simulink model "FuzzyHYPFWMLI"  (R2020b)
settings: Solver=ode23t  StartTime=0.0  StopTime=1  FixedStep=1.0000000100000003E-5  MaxStep=1e-3  RelTol=1e-2  EnableMultiTasking=on
undefined symbols (not defined in the file): c1, c2, c3, c4, c5, c6, DiscIntNeverNeededParam, FC1, FC2, idq1, idq2, PV10k1, PV10k2, PV10k3, R, WM1
libraries: powerlib x93, powerlib_meascontrol x9, fuzblock x8, powerlib_extras x6, re_lib x3, electricdrivelib x2, pid_lib x1
(part 1 of 2)
settings Model: Creator=yaju
settings SolverCC: ZeroCrossControl=DisableAll  AlgebraicLoopSolver=LineSearch
settings DataIOCC: ReturnWorkspaceOutputs=off
settings OptimizationCC: LifeSpan=inf
settings DebuggingCC: SFUnexpectedBacktrackingDiag=warning  SFNoUnconditionalDefaultTransitionDiag=warning  SFExecutionAtInitializationDiag=none  ArithmeticOperatorsInVariantConditions=warning
settings SFSimCC: SimUseLocalCustomCode=off  CustomCodeUndefinedFunction=UseInterfaceOnly
settings RTWCC: RTWUseLocalCustomCode=off
settings CodeAppCC: StateflowObjectComments=on
settings GRTTargetCC: TargetLangStandard=C89/C90 (ANSI)
settings ConfigComp: CovMetricSettings=dw  CovSaveCumulativeToWorkspaceVar=on  CovSaveSingleToWorkspaceVar=on  CovExternalEMLEnable=off  CovBoundaryAbsTol=1.0e-5
settings SimscapeCC: SimscapeNormalizeSystem=off

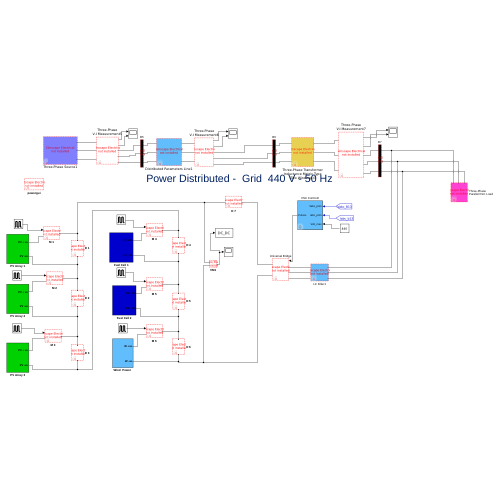
[thumbnail: Simulink's stored preview of the top-level diagram]
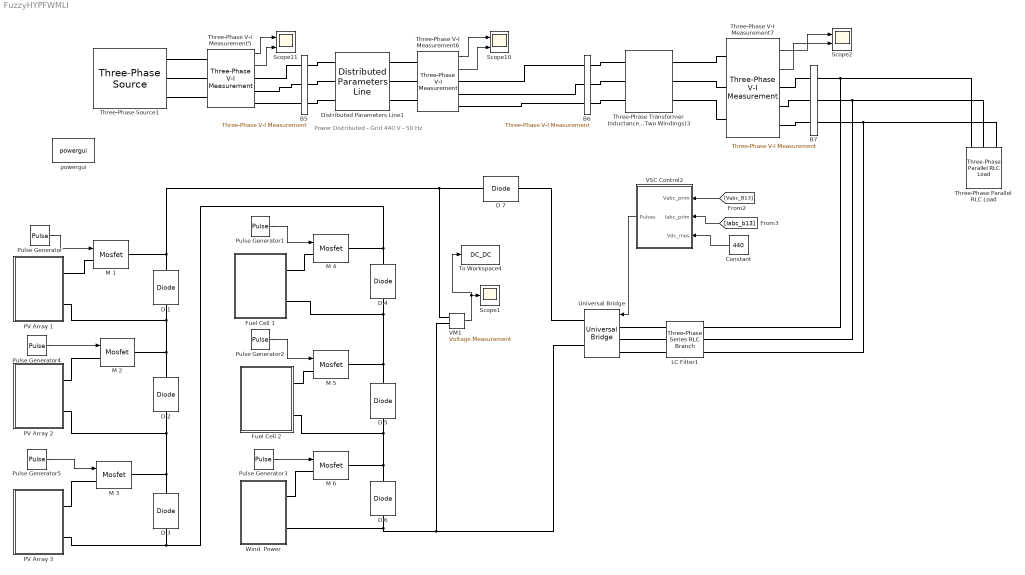
== system FuzzyHYPFWMLI ==
  note: Power Distributed - Grid 440 V - 50 Hz
  B5 : powerlib/Measurements/Three-Phase V-I Measurement  VoltageMeasurement=no  SetLabelV=off  LabelV=Vabc_B12  Vpu=off  VpuLL=off  CurrentMeasurement=no  SetLabelI=off  LabelI=A1  Ipu=off  Pbase=100e6  Vbase=25e3  OutputType=Magnitude  PhasorSimulation=off  PSBequivalent=0
  B6 : powerlib/Measurements/Three-Phase V-I Measurement  VoltageMeasurement=no  SetLabelV=off  LabelV=Vabc_B12  Vpu=off  VpuLL=off  CurrentMeasurement=no  SetLabelI=off  LabelI=A1  Ipu=off  Pbase=100e6  Vbase=440  OutputType=Magnitude  PhasorSimulation=off  PSBequivalent=0
  B7 : powerlib/Measurements/Three-Phase V-I Measurement  VoltageMeasurement=phase-to-ground  SetLabelV=on  LabelV=Vabc_B13  Vpu=off  VpuLL=off  CurrentMeasurement=yes  SetLabelI=on  LabelI=Iabc_b13  Ipu=off  Pbase=100e6  Vbase=440  OutputType=Magnitude  PhasorSimulation=off  PSBequivalent=0
  Constant : Constant  Value=440
  D {1..7} (7 alike) : powerlib/Power Electronics/Diode  Ron=0.00001  Lon=0  Vf=0  IC=0  UseSnubber=off  Rs=inf  Cs=0  Measurements=off
  Distributed Parameters Line1 : powerlib/Elements/Distributed Parameters Line  Phases=3  Frequency=50  Resistance=[0.01273 0.3864]  Inductance="[0.9337e-3  4.1264e-3]"  Capacitance=[12.74e-9 7.751e-9]  Length=100  x1=[-0.00057 -1.30078134445774e-10 0 0;-0.00056 -1.32375687672932e-10 0 0;-0.00055 -1.34671934405495e-10 0 0;-0.00054 -1.36966851980434e-10 0 0;-0.00053 -1.3926041774784e-10 0 0;-0.00052 -1.41552609071144e-10 0 0;-0.00051 -1.43843403327344e-10 0 0;-0.0005 -1.46132777907226e-10 0 0;-0.00049 -1.48420710215585e-10 0 0;-0.00048 -1.50707177671454e-10 0 0;-0.00047 -1.52992157708323e-10 0 0;-0.00046 -1.55275627774361e-10 0 0;-0.00045 -1.5755756533264e-10 0 0;-0.00044 -1.59837947861357e-10 0 0;-0.00043 -1.62116752854058e-10 0 0;-0.00042 -1.64393957819858e-10 0 0;-0.00041 -1.66669540283663e-10 0 0;-0.0004 -1.68943477786392e-10 0 0;-0.00039 -1.71215747885201e-10 0 0;-0.00038 -1.73486328153701e-10 0 0;-0.00037 -1.75755196182181e-10 0 0;-0.00036 -1.7802232957783e-10 0 0;-0.00035 -1.80287705964957e-10 25764.9329895724 -59181.0282967784;-0.00034 -1.82551302985211e-10 25950.7282227276 -59099.7934592953;-0.00033 -1.84813098297803e-10 26136.267332672 -59017.9753307104;-0.00032 -1.87073069579727e-10 26321.5484882094 -58935.5747185355;-0.00031 -1.89331194525979e-10 26506.5698606897 -58852.5924360314;-0.0003 -1.91587450849777e-10 26691.3296240266 -58769.0293021996;-0.00029 -1.93841816282782e-10 26875.8259547158 -58684.8861417747;-0.00028 -1.96094268575318e-10 27060.0570318531 -58600.1637852156;-0.00027 -1.98344785496589e-10 27244.0210371521 -58514.8630686978;-0.00026 -2.00593344834902e-10 27427.7161549622 -58428.9848341049;-0.00025 -2.02839924397885e-10 27611.140572287 -58342.5299290204;-0.00024 -2.05084502012703e-10 27794.2924788014 -58255.4992067194;-0.00023 -2.07327055526283e-10 27977.17006687 -58167.8935261599;-0.00022 -2.09567562805526e-10 28159.7715315649 -58079.7137519746;-0.00021 -2.1180600173753e-10 28342.0950706833 -57990.9607544623;-0.0002 -2.14042350229806e-10 28524.1388847655 -57901.6354095792;-0.00019 -2.16276586210498e-10 28705.9011771127 -57811.7385989305;-0.00018 -2.18508687628599e-10 28887.3801538042 -57721.2712097614;-0.00017 -2.20738632454168e-10 29068.5740237159 -57630.2341349485;-0.00016 -2.2296639867855e-10 29249.4809985375 -57538.6282729909;-0.00015 -2.25191964314593e-10 29430.0992927901 -57446.4545280015;-0.00014 -2.27415307396862e-10 29610.4271238441 -57353.713809698;-0.00013 -2.29636405981858e-10 29790.4627119366 -57260.4070333939;-0.00012 -2.31855238148235e-10 29970.2042801891 -57166.5351199893;-0.00011 -2.34071781997015e-10 30149.6500546247 -57072.0989959621;-0.0001 -2.36286015651805e-10 30328.7982641862 -56977.0995933588;-9e-05 -2.38497917259013e-10 30507.6471407531 -56881.537849785;-8e-05 -2.40707464988064e-10 30686.1949191592 -56785.4147083967;-7e-05 -2.42914637031613e-10 30864.4398372099 -56688.7311178905;-6e-05 -2.45119411605762e-10 31042.3801356999 -56591.4880324942;-5e-05 -2.47321766950278e-10 31220.0140584302 -56493.686411958;-4e-05 -2.49521681328802e-10 31397.3398522259 -56395.3272215443;-3e-05 -2.51719133029067e-10 31574.3557669528 -56296.4114320187;-2e-05 -2.53914100363113e-10 31751.0600555354 -56196.94001964;-1e-05 -2.56106561667497e-10 31927.4509739736 -56096.9139661509]  x2=[-0.00057 -2.06840243965178e-10 0 0;-0.00056 -2.16852614078585e-10 0 0;-0.00055 -2.26862843944237e-10 0 0;-0.00054 -2.36870834765207e-10 0 0;-0.00053 -2.46876487766668e-10 0 0;-0.00052 -2.56879704196862e-10 0 0;-0.00051 -2.66880385328082e-10 0 0;-0.0005 -2.76878432457643e-10 0 0;-0.00049 -2.86873746908856e-10 0 0;-0.00048 -2.96866230032002e-10 0 0;-0.00047 -3.06855783205308e-10 0 0;-0.00046 -3.16842307835916e-10 0 0;-0.00045 -3.2682570536086e-10 0 0;-0.00044 -3.36805877248038e-10 0 0;-0.00043 -3.46782724997181e-10 0 0;-0.00042 -3.5675615014083e-10 0 0;-0.00041 -3.66726054245305e-10 0 0;-0.0004 -3.76692338911678e-10 0 0;-0.00039 -3.86654905776744e-10 0 0;-0.00038 -3.96613656513988e-10 0 0;-0.00037 -4.06568492834561e-10 0 0;-0.00036 -4.16519316488249e-10 0 0;-0.00035 -4.26466029264439e-10 25871.2785310306 -59545.5888484983;-0.00034 -4.36408532993091e-10 26058.2185382591 -59464.0181181603;-0.00033 -4.46346729545707e-10 26244.9013613908 -59381.8605019701;-0.00032 -4.56280520836301e-10 26431.3251579416 -59299.1168107902;-0.00031 -4.66209808822362e-10 26617.4880879838 -59215.7878612673;-0.0003 -4.76134495505826e-10 26803.3883141644 -59131.8744758247;-0.00029 -4.86054482934043e-10 26989.0240017234 -59047.3774826534;-0.00028 -4.95969673200741e-10 27174.3933185114 -58962.2977157048;-0.00027 -5.05879968446996e-10 27359.4944350081 -58876.6360146818;-0.00026 -5.15785270862194e-10 27544.3255243402 -58790.3932250308;-0.00025 -5.25685482685e-10 27728.8847622995 -58703.5701979333;-0.00024 -5.3558050620432e-10 27913.1703273608 -58616.1677902975;-0.00023 -5.45470243760266e-10 28097.1804006999 -58528.18686475;-0.00022 -5.55354597745121e-10 28280.9131662118 -58439.6282896269;-0.00021 -5.65233470604303e-10 28464.3668105282 -58350.4929389656;-0.0002 -5.75106764837323e-10 28647.5395230356 -58260.781692496;-0.00019 -5.84974382998755e-10 28830.4294958935 -58170.495435632;-0.00018 -5.9483622769919e-10 29013.0349240516 -58079.6350594623;-0.00017 -6.04692201606202e-10 29195.354005268 -57988.2014607424;-0.00016 -6.14542207445309e-10 29377.384940127 -57896.1955418848;-0.00015 -6.24386148000929e-10 29559.1259320568 -57803.6182109509;-0.00014 -6.34223926117344e-10 29740.5751873472 -57710.4703816414;-0.00013 -6.44055444699654e-10 29921.7309151672 -57616.752973288;-0.00012 -6.5388060671474e-10 30102.5913275829 -57522.4669108435;-0.00011 -6.63699315192221e-10 30283.1546395752 -57427.6131248734;-0.0001 -6.73511473225407e-10 30463.419069057 -57332.1925515463;-9e-05 -6.8331698397226e-10 30643.3828368911 -57236.2061326245;-8e-05 -6.93115750656347e-10 30823.0441669079 -57139.6548154555;-7e-05 -7.02907676567797e-10 31002.4012859225 -57042.5395529616;-6e-05 -7.12692665064255e-10 31181.4524237526 -56944.8613036313;-5e-05 -7.22470619571835e-10 31360.1958132358 -56846.6210315096;-4e-05 -7.32241443586072e-10 31538.6296902468 -56747.8197061882;-3e-05 -7.42005040672879e-10 31716.7522937155 -56648.4583027963;-2e-05 -7.51761314469494e-10 31894.5618656437 -56548.5378019908;-1e-05 -7.61510168685434e-10 32072.0566511226 -56448.0591899468]  x3=[-0.00057 1.68975280202087e-11 0 0;-0.00056 1.68765883509604e-11 0 0;-0.00055 1.68554821165985e-11 0 0;-0.00054 1.68342095254328e-11 0 0;-0.00053 1.68127707874154e-11 0 0;-0.00052 1.67911661141379e-11 0 0;-0.00051 1.67693957188297e-11 0 0;-0.0005 1.67474598163559e-11 0 0;-0.00049 1.67253586232149e-11 0 0;-0.00048 1.67030923575366e-11 0 0;-0.00047 1.668066123908e-11 0 0;-0.00046 1.66580654892313e-11 0 0;-0.00045 1.66353053310013e-11 0 0;-0.00044 1.66123809890236e-11 0 0;-0.00043 1.65892926895523e-11 0 0;-0.00042 1.65660406604595e-11 0 0;-0.00041 1.65426251312333e-11 0 0;-0.0004 1.65190463329757e-11 0 0;-0.00039 1.64953044983997e-11 0 0;-0.00038 1.64713998618278e-11 0 0;-0.00037 1.6447332659189e-11 0 0;-0.00036 1.64231031280169e-11 0 0;-0.00035 1.63987115074472e-11 70.7662938963626 -227.139574442311;-0.00034 1.63741580382154e-11 71.479523523603 -226.916135051034;-0.00033 1.63494429626542e-11 72.1920476768036 -226.690456089114;-0.00032 1.63245665246915e-11 72.9038593236387 -226.462539783912;-0.00031 1.62995289698478e-11 73.6149514388149 -226.232388384868;-0.0003 1.62743305452334e-11 74.3253170041398 -226.000004163484;-0.00029 1.62489714995469e-11 75.0349490085923 -225.7653894133;-0.00028 1.62234520830715e-11 75.7438404483909 -225.528546449867;-0.00027 1.61977725476738e-11 76.4519843270633 -225.28947761073;-0.00026 1.61719331468004e-11 77.1593736555153 -225.048185255402;-0.00025 1.61459341354757e-11 77.8660014520998 -224.804671765341;-0.00024 1.61197757702994e-11 78.5718607426858 -224.558939543928;-0.00023 1.60934583094441e-11 79.276944560727 -224.310991016439;-0.00022 1.60669820126525e-11 79.9812459473307 -224.060828630027;-0.00021 1.60403471412349e-11 80.6847579513268 -223.808454853693;-0.0002 1.60135539580668e-11 81.3874736293355 -223.553872178265;-0.00019 1.5986602727586e-11 82.089386045837 -223.297083116371;-0.00018 1.59594937157904e-11 82.7904882732391 -223.038090202415;-0.00017 1.59322271902349e-11 83.4907733919458 -222.776895992553;-0.00016 1.59048034200292e-11 84.1902344904257 -222.513503064667;-0.00015 1.58772226758347e-11 84.8888646652801 -222.247914018337;-0.00014 1.58494852298623e-11 85.5866570213113 -221.980131474821;-0.00013 1.58215913558694e-11 86.2836046715904 -221.710158077025;-0.00012 1.57935413291572e-11 86.9797007375256 -221.437996489476;-0.00011 1.57653354265682e-11 87.6749383489296 -221.1636493983;-0.0001 1.57369739264833e-11 88.3693106440878 -220.887119511192;-9e-05 1.5708457108819e-11 89.0628107698262 -220.60840955739;-8e-05 1.56797852550248e-11 89.7554318815784 -220.327522287649;-7e-05 1.56509586480804e-11 90.4471671434536 -220.044460474212;-6e-05 1.56219775724926e-11 91.1380097283041 -219.759226910787;-5e-05 1.5592842314293e-11 91.8279528177925 -219.471824412512;-4e-05 1.55635531610349e-11 92.5169896024591 -219.182255815935;-3e-05 1.55341104017903e-11 93.2051132817889 -218.89052397898;-2e-05 1.55045143271474e-11 93.892317064279 -218.596631780923;-1e-05 1.54747652292076e-11 94.5785941675056 -218.300582122362]  x4=[-0.00057 -1.66555281463013e-11 0 0;-0.00056 -1.6651971200068e-11 0 0;-0.00055 -1.66482499056017e-11 0 0;-0.00054 -1.664436429963e-11 0 0;-0.00053 -1.66403144205023e-11 0 0;-0.00052 -1.66361003081891e-11 0 0;-0.00051 -1.66317220042822e-11 0 0;-0.0005 -1.66271795519937e-11 0 0;-0.00049 -1.66224729961556e-11 0 0;-0.00048 -1.66176023832198e-11 0 0;-0.00047 -1.66125677612573e-11 0 0;-0.00046 -1.66073691799577e-11 0 0;-0.00045 -1.6602006690629e-11 0 0;-0.00044 -1.65964803461968e-11 0 0;-0.00043 -1.65907902012038e-11 0 0;-0.00042 -1.65849363118095e-11 0 0;-0.00041 -1.65789187357894e-11 0 0;-0.0004 -1.65727375325346e-11 0 0;-0.00039 -1.6566392763051e-11 0 0;-0.00038 -1.6559884489959e-11 0 0;-0.00037 -1.65532127774925e-11 0 0;-0.00036 -1.65463776914988e-11 0 0;-0.00035 -1.65393792994372e-11 95.5719621574451 -220.194613156224;-0.00034 -1.65322176703792e-11 96.2632511702535 -219.893278859941;-0.00033 -1.65248928750071e-11 96.9535901036358 -219.589774305771;-0.00032 -1.65174049856138e-11 97.6429721442256 -219.28410248918;-0.00031 -1.65097540761015e-11 98.3313904881003 -218.976266427026;-0.0003 -1.65019402219818e-11 99.0188383408489 -218.666269157526;-0.00029 -1.64939635003742e-11 99.7053089176387 -218.354113740229;-0.00028 -1.64858239900057e-11 100.390795443282 -218.039803255983;-0.00027 -1.647752177121e-11 101.075291152304 -217.723340806905;-0.00026 -1.64690569259267e-11 101.758789289008 -217.404729516351;-0.00025 -1.64604295377004e-11 102.441283107543 -217.083972528887;-0.00024 -1.64516396916798e-11 103.122765871971 -216.761073010254;-0.00023 -1.64426874746174e-11 103.803230856332 -216.436034147341;-0.00022 -1.64335729748677e-11 104.482671344712 -216.10885914815;-0.00021 -1.64242962823872e-11 105.161080631307 -215.779551241765;-0.0002 -1.64148574887332e-11 105.838452020492 -215.448113678324;-0.00019 -1.64052566870628e-11 106.514778826884 -215.11454972898;-0.00018 -1.63954939721319e-11 107.19005437541 -214.778862685876;-0.00017 -1.63855694402946e-11 107.864272001374 -214.441055862106;-0.00016 -1.63754831895021e-11 108.53742505052 -214.101132591689;-0.00015 -1.63652353193015e-11 109.209506879099 -213.759096229529;-0.00014 -1.63548259308353e-11 109.880510853935 -213.414950151388;-0.00013 -1.63442551268398e-11 110.55043035249 -213.068697753847;-0.00012 -1.63335230116447e-11 111.219258762927 -212.720342454279;-0.00011 -1.63226296911716e-11 111.886989484182 -212.36988769081;-0.0001 -1.63115752729331e-11 112.553615926022 -212.017336922287;-9e-05 -1.63003598660319e-11 113.219131509111 -211.662693628242;-8e-05 -1.62889835811596e-11 113.883529665082 -211.305961308864;-7e-05 -1.62774465305954e-11 114.546803836591 -210.947143484955;-6e-05 -1.62657488282055e-11 115.20894747739 -210.586243697902;-5e-05 -1.62538905894414e-11 115.86995405239 -210.223265509642;-4e-05 -1.62418719313391e-11 116.529817037722 -209.858212502621;-3e-05 -1.62296929725179e-11 117.188529920804 -209.491088279766;-2e-05 -1.62173538331794e-11 117.846086200408 -209.121896464445;-1e-05 -1.62048546351057e-11 118.502479386716 -208.750640700432]  x5=0.000565541566995743  V1=[0 0 0 6.811e-10 6.455e+04 6.455e+04;0 0 0 314.2 314.2 314.2;1.571 1.571 1.571 -2.987 0.4122 -1.159]  V2=[0 0 0 3.037e-09 6.492e+04 6.492e+04;0 0 0 314.2 314.2 314.2;1.571 1.571 1.571 -3.09 0.4115 -1.159]  I1=[0 0 0 1.726e-11 237.9 237.9;0 0 0 314.2 314.2 314.2;1.571 1.571 1.571 1.917 0.3036 -1.267]  I2=[0 0 0 1.627e-11 240 240;0 0 0 314.2 314.2 314.2;1.571 1.571 1.571 -1.497 0.4111 -1.16]  nHarmo=2  Measurements=None
      settings: SourceProductName=Simscape Power Systems
  Fuel Cell 1 : Subsystem
  Fuel Cell 2 : Subsystem
  LC Filter1 : powerlib/Elements/Three-Phase Series RLC Branch  LConnTagsString=A|B|C  RConnTagsString=A|B|C  BranchType=LC  Resistance=500e-6*377/50/2  Inductance=2e-2  Capacitance=550e-6  Measurements=None
  M {1..6} (6 alike) : powerlib/Power Electronics/Mosfet  Ron=0.1  Lon=0  Rd=0.01  Vfd=0  IC=0  Rs=1e5  Cs=inf  Measurements=off
  PV Array 1 : Subsystem
  PV Array 2 : Subsystem
  PV Array 3 : Subsystem
  Pulse Generator : DiscretePulseGenerator  PulseType=Time based  Period=0.01  PulseWidth=99.999999
  Pulse Generator1 : DiscretePulseGenerator  PulseType=Time based  Period=0.01  PulseWidth=51  PhaseDelay=0.00249
  Pulse Generator2 : DiscretePulseGenerator  PulseType=Time based  Period=0.01  PulseWidth=34  PhaseDelay=0.00333
  Pulse Generator3 : DiscretePulseGenerator  PulseType=Time based  Period=0.01  PulseWidth=17  PhaseDelay=0.0041
  Pulse Generator4 : DiscretePulseGenerator  PulseType=Time based  Period=0.01  PulseWidth=85  PhaseDelay=0.000833
  Pulse Generator5 : DiscretePulseGenerator  PulseType=Time based  Period=0.01  PulseWidth=68  PhaseDelay=0.00166
  Scope1 : Scope
  Scope10 : Scope  NumInputPorts=2
  Scope11 : Scope  NumInputPorts=2
  Scope2 : Scope  NumInputPorts=2
  Three-Phase Parallel RLC Load : powerlib/Elements/Three-Phase Parallel RLC Load  LConnTagsString=A|B|C  Configuration=Y (grounded)  NominalVoltage=220  Vabc=[1e3 1e3 1e3]  Vabcp=[1e3 1e3 1e3]  NominalFrequency=50  UnbalancedPower=off  ActivePower=50e3  InductivePower=1000  CapacitivePower=0  Pabc=[10e3 9e3 11e3]  QLabc=[100 90 110]  QCabc=[100 90 110]  Pabcp=[10e3 9e3 11e3]  QLabcp=[100 90 110]  QCabcp=[100 90 110]  Measurements=None  LoadType=constant Z
  Three-Phase V-I Measurement5 : powerlib/Measurements/Three-Phase V-I Measurement  VoltageMeasurement=phase-to-ground  SetLabelV=off  LabelV=Vabc  Vpu=off  VpuLL=off  CurrentMeasurement=yes  SetLabelI=off  LabelI=Iabc  Ipu=off  Pbase=100e6  Vbase=500e3  OutputType=Complex  PhasorSimulation=off  PSBequivalent=0
  Three-Phase V-I Measurement6 : powerlib/Measurements/Three-Phase V-I Measurement  VoltageMeasurement=phase-to-ground  SetLabelV=off  LabelV=Vabc  Vpu=off  VpuLL=off  CurrentMeasurement=yes  SetLabelI=off  LabelI=Iabc  Ipu=off  Pbase=100e6  Vbase=500e3  OutputType=Complex  PhasorSimulation=off  PSBequivalent=0
  Three-Phase V-I Measurement7 : powerlib/Measurements/Three-Phase V-I Measurement  VoltageMeasurement=phase-to-ground  SetLabelV=off  LabelV=Vabc_b1  Vpu=off  VpuLL=off  CurrentMeasurement=yes  SetLabelI=off  LabelI=Iabc_b1  Ipu=off  Pbase=100e6  Vbase=500e3  OutputType=Complex  PhasorSimulation=off  PSBequivalent=0
  Three-Phase Source1 : powerlib/Electrical Sources/Three-Phase Source  InternalConnection=Yg  VoltagePhases=off  Voltage=63510.4  PhaseAngle=0  Voltage_phases=[25e3 25e3 25e3]/sqrt(3)  PhaseAngles_phases=[0 -120 +120]  Frequency=50  NonIdealSource=on  SpecifyImpedance=on  Resistance=0.8929  Inductance=16.58e-3  ShortCircuitLevel=100e6  BaseVoltage=63510.4  XRratio=7  BusType=swing  Pref=0  Qref=0  Prefabc=[10e3, 10e3, 10e3]  Qrefabc=[0, 0, 0]  Qmin=-inf  Qmax=inf
  Three-Phase Transformer Inductance Matrix Type (Two Windings)3 : powerlib/Elements/Three-Phase Transformer Inductance Matrix Type (Two Windings)  CoreType=Three-limb or five-limb core  Winding1Connection=Yg  Winding2Connection=Yg  AutoTransformer=off  Measurements=None  NominalPower=[100e3 50]  VLLnom=[63510.4 254.03]  WindingResistances=[0.01 0.01]  NoLoadIexcPos=2  NoLoadPlossPos=1000  ShortCircuitReactancePos=0.06  ShortCircuitReactancePosAuto=0.06  NoLoadIexcZero=100  NoLoadPlossZero=1500  ShortCircuitReactanceZero=0.03  ShortCircuitReactanceZeroAuto=0.03
      settings: SourceProductName=Simscape Power Systems
  To Workspace4 : ToWorkspace  VariableName=DC_DC  SaveFormat=Timeseries  SampleTime=-1
  Universal Bridge : powerlib/Power Electronics/Universal Bridge  Arms=3  SnubberResistance=1e5  SnubberCapacitance=inf  Device=MOSFET / Diodes  Ron=1e-3  Lon=0  ForwardVoltages="[  0  0  ]"  ForwardVoltage=0  GTOparameters=[ 10e-6 , 20e-6 ]  IGBTparameters=[ 1e-6 , 2e-6 ]  Measurements=None  Measurements_2=None  converterType=Rectifier
  VM1 : powerlib/Measurements/Voltage Measurement  PhasorSimulation=off  OutputType=Complex  PSBequivalent=0
  VSC Control2 : Subsystem  mask(VSC Main Controller){nom=[ 100e3  50 ], Vnom=[ 25e3 260 ], Vnom_dc=220, RLxfo=[0.002  0.06 ], RLchoke=[2e-3  250e-6  ], K_VDCreg=[7  800], K_Ireg=[0.3 20], Ts=1e-6}
      mask prompts: nom "Nominal power and frequency [ Pnom(VA)  Fnom(Hz) ]:"; Vnom "Nominal primary and secondary voltages (Vrms LL) [ Vnom_prim   Vnom_sec ]:"; Vnom_dc "Nominal DC bus voltage (V):"; RLxfo "Total transformer leakage impedance (pu/Pnom) [ Rxfo  Lxf ]"; RLchoke "Choke impedance [ R(ohm) L(H) ]"; K_VDCreg "VDC regultator gains [ Kp  Ki ]:"; K_Ireg "Current regulator gains [ Kp  Ki ]:"; Ts "Sample time"
      mask init:
      | Pnom=nom(1);
      | Fnom=nom(2);
      | Vnom_prim=Vnom(1);
      | Vnom_sec=Vnom(2);
      | Zbase=Vnom_sec^2/Pnom;
      | Rtot_pu=RLxfo(1) + RLchoke(1)/Zbase;
      | Ltot_pu=RLxfo(2) + RLchoke(2)/(Zbase/(2*pi*Fnom));
      | Kp_VDCreg=K_VDCreg(1);
      | Ki_VDCreg=K_VDCreg(2);
      | Kp_Ireg=K_Ireg(1);
      | Ki_Ireg=K_Ireg(2);
      | Vdc_ref=Vnom_dc;
      | % Used to determine initial value of Boost Control (MPPT)
      | assignin('base','Vdc_ref_Inv',Vdc_ref);
  "Wind  Power " : Subsystem
  powergui : powerlib/powergui  Priority=1  SimulationMode=Discrete  SampleTime=0.00001  frequency=60  Iterations=50  frequencyindice=0  Pbase=100e6  ErrMax=1e-4  UnitsV=kV  UnitsW=MW  buscounter=0  FunctionMessages=off  echomessages=off  EnableUseOfTLC=off  CurrentSourceSwitches=off  DisableSnubberDevices=off  DisableRonSwitches=off  DisableVfSwitches=off  DisplayEquations=off  SolverType=Tustin/Backward Euler (TBE)  Interpol=off  ExternalGateDelay=off  methode=off  Ts=100  x0status=blocks  SPID=off  SwTol=0  HookPort=off  RestoreLinks=warning  ResistiveCurrentMeasurement=off  Frange=[0:2:500]  Ylog=off  Xlog=on  ShowGrid=off  save=off  variable=ZData  structure=DG  ZoomFFT=off  StartTime=0.012  cycles=1  DisplayStyle=1  fundamental=50  FreqAxis=on  MaxFrequency=1000  frequencyindicesteady=1  RmsSteady=1  display=off
  wires:
  Pulse Generator/1 -> M 1/1
  Pulse Generator4/1 -> M 2/1
  Pulse Generator5/1 -> M 3/1
  VM1/1 -> To Workspace4/1, Scope1/1
  Pulse Generator3/1 -> M 6/1
  Pulse Generator2/1 -> M 5/1
  Pulse Generator1/1 -> M 4/1
  Three-Phase V-I Measurement6/1 -> Scope10/1
  Three-Phase V-I Measurement5/2 -> Scope11/2
  Three-Phase V-I Measurement7/1 -> Scope2/1
  Three-Phase V-I Measurement7/2 -> Scope2/2
  Three-Phase V-I Measurement5/1 -> Scope11/1
  Three-Phase V-I Measurement6/2 -> Scope10/2
  [Vabc_B13] -> VSC Control2/1(Vabc_prim)
  [Iabc_b13] -> VSC Control2/2(Iabc_prim)
  VSC Control2/1(Pulses) -> Universal Bridge/1
  Constant/1 -> VSC Control2/3(Vdc_mes)
  connections:
  D 1/RConn1 -- D 7/LConn1 -- VM1/LConn1 -- M 1/RConn1
  M 2/RConn1 -- D 2/RConn1 -- PV Array 1/RConn2 -- D 1/LConn1
  D 2/LConn1 -- PV Array 2/RConn2 -- D 3/RConn1 -- M 3/RConn1
  D 3/LConn1 -- D 4/RConn1 -- M 4/RConn1 -- PV Array 3/RConn2
  D 4/LConn1 -- Fuel Cell 1/RConn2 -- D 5/RConn1 -- M 5/RConn1
  D 5/LConn1 -- Fuel Cell 2/RConn2 -- D 6/RConn1 -- M 6/RConn1
  VM1/LConn2 -- Universal Bridge/RConn2 -- D 6/LConn1 -- "Wind  Power "/RConn2
  M 3/LConn1 -- PV Array 3/RConn1
  M 4/LConn1 -- Fuel Cell 1/RConn1
  M 1/LConn1 -- PV Array 1/RConn1
  M 6/LConn1 -- "Wind  Power "/RConn1
  M 2/LConn1 -- PV Array 2/RConn1
  M 5/LConn1 -- Fuel Cell 2/RConn1
  Three-Phase V-I Measurement7/RConn2 -- B7/RConn2
  Three-Phase V-I Measurement7/LConn3 -- Three-Phase Transformer Inductance Matrix Type (Two Windings)3/RConn3
  B6/RConn1 -- Three-Phase V-I Measurement6/RConn1
  Distributed Parameters Line1/LConn1 -- B5/LConn1
  Distributed Parameters Line1/LConn2 -- B5/LConn2
  Three-Phase Transformer Inductance Matrix Type (Two Windings)3/LConn2 -- B6/LConn2
  Three-Phase Source1/RConn2 -- Three-Phase V-I Measurement5/LConn2
  Three-Phase V-I Measurement6/LConn3 -- Distributed Parameters Line1/RConn3
  B7/LConn3 -- Three-Phase Parallel RLC Load/LConn3 -- LC Filter1/RConn3
  B6/RConn2 -- Three-Phase V-I Measurement6/RConn2
  B7/LConn2 -- Three-Phase Parallel RLC Load/LConn2 -- LC Filter1/RConn2
  Three-Phase V-I Measurement7/RConn3 -- B7/RConn3
  B5/RConn2 -- Three-Phase V-I Measurement5/RConn2
  Three-Phase Source1/RConn1 -- Three-Phase V-I Measurement5/LConn1
  Three-Phase V-I Measurement7/RConn1 -- B7/RConn1
  B5/RConn1 -- Three-Phase V-I Measurement5/RConn1
  B6/RConn3 -- Three-Phase V-I Measurement6/RConn3
  B7/LConn1 -- Three-Phase Parallel RLC Load/LConn1 -- LC Filter1/RConn1
  Three-Phase Transformer Inductance Matrix Type (Two Windings)3/LConn1 -- B6/LConn1
  Three-Phase V-I Measurement6/LConn2 -- Distributed Parameters Line1/RConn2
  Three-Phase Source1/RConn3 -- Three-Phase V-I Measurement5/LConn3
  Distributed Parameters Line1/LConn3 -- B5/LConn3
  Three-Phase Transformer Inductance Matrix Type (Two Windings)3/LConn3 -- B6/LConn3
  Three-Phase V-I Measurement7/LConn1 -- Three-Phase Transformer Inductance Matrix Type (Two Windings)3/RConn1
  Three-Phase V-I Measurement6/LConn1 -- Distributed Parameters Line1/RConn1
  B5/RConn3 -- Three-Phase V-I Measurement5/RConn3
  Three-Phase V-I Measurement7/LConn2 -- Three-Phase Transformer Inductance Matrix Type (Two Windings)3/RConn2
  LC Filter1/LConn3 -- Universal Bridge/LConn3
  LC Filter1/LConn1 -- Universal Bridge/LConn1
  LC Filter1/LConn2 -- Universal Bridge/LConn2
  D 7/RConn1 -- Universal Bridge/RConn1

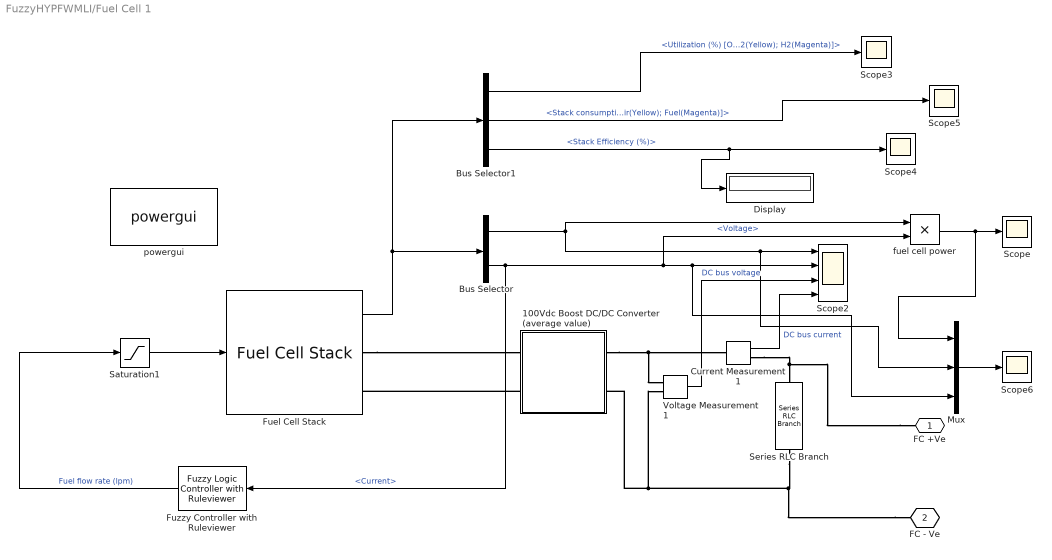
== system FuzzyHYPFWMLI/Fuel Cell 1 ==
  100Vdc Boost DC/DC Converter (average value) : Subsystem
  Bus Selector : BusSelector  OutputSignals=Voltage,Current
  Bus Selector1 : BusSelector  OutputSignals=Utilization (%) [O2(Yellow); H2(Magenta)],Stack consumption (lpm) [Air(Yellow); Fuel(Magenta)],Stack Efficiency (%)
  Current Measurement1 : powerlib/Measurements/Current Measurement  PhasorSimulation=off  OutputType=Complex  PSBequivalent=0
  Display : Display
  Fuel Cell Stack : electricdrivelib/Extra Sources/Fuel Cell Stack  PresetModel=PEMFC - 6 kW - 45 Vdc  FcType=Proton Exchange Membrane (PEM)  Detailed=Detailed  Eoc=[65,63]  NomVI=[133.3,45]  EndVI=[225,37]  Nc=65  n=55  TOp=65  AirFr=300  SuppPress=[1.5,1]  Comp=[99.95,21,1]  SignX=off  SignY=off  FlowRateH2=on  FlowRateAir=off  SystemTemp=off  SystemPH2=off  SystemPAir=off  FCDyn=on  FC_tau=0  Peak_O2=80  V_Under=10
      settings: SourceProductName=Simscape Power Systems
  Fuzzy Controller with Ruleviewer : fuzblock/Fuzzy Logic  Controller  with Ruleviewer  fismatrix=[FC1]  Ts=0.1
  Mux : Mux  Inputs=3
  Saturation1 : Saturate  UpperLimit=48.9  LowerLimit=48.3  RndMeth=Nearest
  Scope{,3..6} (5 alike) : Scope
  Scope2 : Scope  NumInputPorts=4
  Series RLC Branch : powerlib/Elements/Series RLC Branch  LConnTagsString=__new0  RConnTagsString=__new0  BranchType=RL  Resistance=100*100/6000  Inductance=100*100/6000  SetiL0=off  InitialCurrent=0  Capacitance=1e-6  Setx0=off  InitialVoltage=0  Measurements=None
  Voltage Measurement1 : powerlib/Measurements/Voltage Measurement  PhasorSimulation=off  OutputType=Complex  PSBequivalent=0
  fuel cell power : Product  RndMeth=Zero
  powergui : powerlib/powergui  SimulationMode=Discrete  SampleTime=1e-6  frequency=60  Iterations=50  frequencyindice=0  Pbase=100e6  ErrMax=1e-4  UnitsV=kV  UnitsW=MW  buscounter=0  FunctionMessages=off  echomessages=off  EnableUseOfTLC=off  CurrentSourceSwitches=off  DisableSnubberDevices=off  DisableRonSwitches=off  DisableVfSwitches=off  DisplayEquations=off  SolverType=Tustin/Backward Euler (TBE)  Interpol=off  ExternalGateDelay=off  methode=off  Ts=100  x0status=blocks  SPID=off  SwTol=0  HookPort=off  RestoreLinks=warning  ResistiveCurrentMeasurement=off  Frange=[0:2:500]  Ylog=off  Xlog=on  ShowGrid=off  save=off  variable=ZData  structure=0  ZoomFFT=on  StartTime=0.0  cycles=1  DisplayStyle=1  fundamental=60  FreqAxis=off  MaxFrequency=1000  frequencyindicesteady=1  RmsSteady=1  display=off
  FC +Ve : PMIOPort  Side=Right
  FC - Ve : PMIOPort  Port=2  Side=Right
  wires:
  Saturation1/1 -> Fuel Cell Stack/1
  Voltage Measurement1/1 -> Scope2/3  "DC bus voltage"
  Bus Selector1/2 -> Scope5/1  "<Stack consumption (lpm) [Air(Yellow); Fuel(Magenta)]>"
  Current Measurement1/1 -> Scope2/4  "DC bus current"
  Fuel Cell Stack/1 -> Bus Selector/1, Bus Selector1/1
  Bus Selector1/1 -> Scope3/1  "<Utilization (%) [O2(Yellow); H2(Magenta)]>"
  fuel cell power/1 -> Scope/1, Mux/1
  Bus Selector1/3 -> Scope4/1, Display/1  "<Stack Efficiency (%)>"
  Bus Selector/1 -> fuel cell power/1, Scope2/1, Mux/2  "<Voltage>"
  Mux/1 -> Scope6/1
  Bus Selector/2 -> Scope2/2, Mux/3, fuel cell power/2, Fuzzy Controller with Ruleviewer/1  "<Current>"
  Fuzzy Controller with Ruleviewer/1 -> Saturation1/1  "Fuel flow rate (lpm)"
  connections:
  FC +Ve/RConn1 -- Current Measurement1/RConn1 -- Series RLC Branch/LConn1
  Fuel Cell Stack/RConn1 -- 100Vdc Boost DC/DC Converter (average value)/LConn1
  100Vdc Boost DC/DC Converter (average value)/LConn2 -- Fuel Cell Stack/RConn2
  FC - Ve/RConn1 -- Series RLC Branch/RConn1 -- 100Vdc Boost DC/DC Converter (average value)/RConn2 -- Voltage Measurement1/LConn2
  100Vdc Boost DC/DC Converter (average value)/RConn1 -- Voltage Measurement1/LConn1 -- Current Measurement1/LConn1

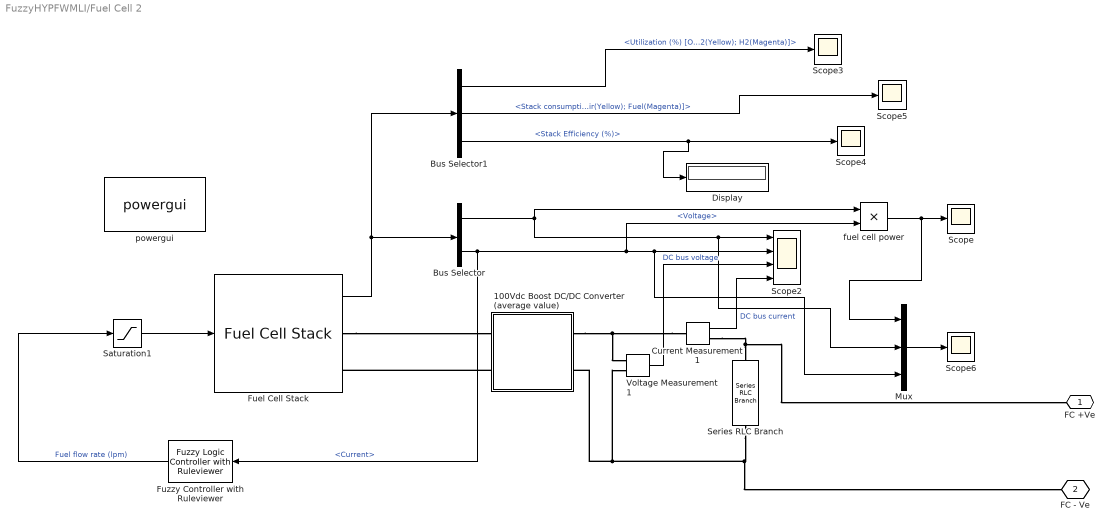
== system FuzzyHYPFWMLI/Fuel Cell 2 ==
  100Vdc Boost DC/DC Converter (average value) : Subsystem
  Bus Selector : BusSelector  OutputSignals=Voltage,Current
  Bus Selector1 : BusSelector  OutputSignals=Utilization (%) [O2(Yellow); H2(Magenta)],Stack consumption (lpm) [Air(Yellow); Fuel(Magenta)],Stack Efficiency (%)
  Current Measurement1 : powerlib/Measurements/Current Measurement  PhasorSimulation=off  OutputType=Complex  PSBequivalent=0
  Display : Display
  Fuel Cell Stack : electricdrivelib/Extra Sources/Fuel Cell Stack  PresetModel=PEMFC - 6 kW - 45 Vdc  FcType=Proton Exchange Membrane (PEM)  Detailed=Detailed  Eoc=[65,63]  NomVI=[133.3,45]  EndVI=[225,37]  Nc=65  n=55  TOp=65  AirFr=300  SuppPress=[1.5,1]  Comp=[99.95,21,1]  SignX=off  SignY=off  FlowRateH2=on  FlowRateAir=off  SystemTemp=off  SystemPH2=off  SystemPAir=off  FCDyn=on  FC_tau=0  Peak_O2=80  V_Under=10
      settings: SourceProductName=Simscape Power Systems
  Fuzzy Controller with Ruleviewer : fuzblock/Fuzzy Logic  Controller  with Ruleviewer  fismatrix=[FC2]  Ts=0.1
  Mux : Mux  Inputs=3
  Saturation1 : Saturate  UpperLimit=48.9  LowerLimit=48.3  RndMeth=Nearest
  Scope{,3..6} (5 alike) : Scope
  Scope2 : Scope  NumInputPorts=4
  Series RLC Branch : powerlib/Elements/Series RLC Branch  LConnTagsString=__new0  RConnTagsString=__new0  BranchType=RL  Resistance=100*100/6000  Inductance=100*100/6000  SetiL0=off  InitialCurrent=0  Capacitance=1e-6  Setx0=off  InitialVoltage=0  Measurements=None
  Voltage Measurement1 : powerlib/Measurements/Voltage Measurement  PhasorSimulation=off  OutputType=Complex  PSBequivalent=0
  fuel cell power : Product  RndMeth=Zero
  powergui : powerlib/powergui  SimulationMode=Discrete  SampleTime=1e-6  frequency=60  Iterations=50  frequencyindice=0  Pbase=100e6  ErrMax=1e-4  UnitsV=kV  UnitsW=MW  buscounter=0  FunctionMessages=off  echomessages=off  EnableUseOfTLC=off  CurrentSourceSwitches=off  DisableSnubberDevices=off  DisableRonSwitches=off  DisableVfSwitches=off  DisplayEquations=off  SolverType=Tustin/Backward Euler (TBE)  Interpol=off  ExternalGateDelay=off  methode=off  Ts=100  x0status=blocks  SPID=off  SwTol=0  HookPort=off  RestoreLinks=warning  ResistiveCurrentMeasurement=off  Frange=[0:2:500]  Ylog=off  Xlog=on  ShowGrid=off  save=off  variable=ZData  structure=0  ZoomFFT=on  StartTime=0.0  cycles=1  DisplayStyle=1  fundamental=60  FreqAxis=off  MaxFrequency=1000  frequencyindicesteady=1  RmsSteady=1  display=off
  FC +Ve : PMIOPort  Side=Right
  FC - Ve : PMIOPort  Port=2  Side=Right
  wires:
  Fuzzy Controller with Ruleviewer/1 -> Saturation1/1  "Fuel flow rate (lpm)"
  Bus Selector/2 -> Fuzzy Controller with Ruleviewer/1, fuel cell power/2, Mux/3, Scope2/2  "<Current>"
  Mux/1 -> Scope6/1
  Bus Selector/1 -> Mux/2, Scope2/1, fuel cell power/1  "<Voltage>"
  Bus Selector1/3 -> Display/1, Scope4/1  "<Stack Efficiency (%)>"
  fuel cell power/1 -> Mux/1, Scope/1
  Bus Selector1/1 -> Scope3/1  "<Utilization (%) [O2(Yellow); H2(Magenta)]>"
  Fuel Cell Stack/1 -> Bus Selector1/1, Bus Selector/1
  Current Measurement1/1 -> Scope2/4  "DC bus current"
  Bus Selector1/2 -> Scope5/1  "<Stack consumption (lpm) [Air(Yellow); Fuel(Magenta)]>"
  Voltage Measurement1/1 -> Scope2/3  "DC bus voltage"
  Saturation1/1 -> Fuel Cell Stack/1
  connections:
  Current Measurement1/LConn1 -- Voltage Measurement1/LConn1 -- 100Vdc Boost DC/DC Converter (average value)/RConn1
  Voltage Measurement1/LConn2 -- 100Vdc Boost DC/DC Converter (average value)/RConn2 -- Series RLC Branch/RConn1 -- FC - Ve/RConn1
  100Vdc Boost DC/DC Converter (average value)/LConn2 -- Fuel Cell Stack/RConn2
  Fuel Cell Stack/RConn1 -- 100Vdc Boost DC/DC Converter (average value)/LConn1
  Series RLC Branch/LConn1 -- Current Measurement1/RConn1 -- FC +Ve/RConn1

== system FuzzyHYPFWMLI/PV Array 1 ==
  note: Fuzzy Based MPPT Controller for 10 kW PV System
  Boost Converter with Fuzzy Controller : Subsystem
  Demux : Demux  Outputs=5
  IRR 2 : powerlib_extras/Control  Blocks/Timer  t=[0 0.05 0.1 0.15 0.2 ]  e=[250 500 750 1000 1000]
  PV Array : re_lib/Solar/PV Array  Npar=6  Nser=9  PlotType=array @ 25 deg.C & specified irradiances  S_vec="[ 1000  500  100 ]"  Temp_C_vec="[ 45 25  ]"  ModuleName=BP Solar SX3200W  PlotWhenSelected=off  Pm=199.92  Ncell=50  Voc=30.8  Isc=8.7  Vm=24.5  Im=8.16  beta_Voc_pc=-0.33  alpha_Isc_pc=0.1  beta_Voc=-0.10164  alpha_Isc=0.0087  IL=8.7449  I0=1.0576e-10  nI=0.95448  Rsh=190.2563  Rs=0.32982  BAL=off  Tc=1e-6  Tfilter=5e-5
  Scope : Scope
  Scope1 : Scope
  Scope2 : Scope  NumInputPorts=3
  Scope5 : Scope  NumInputPorts=5
  "Temp " : Constant  Value=25
  Voltage Measurement : powerlib/Measurements/Voltage Measurement  PhasorSimulation=off  OutputType=Complex  PSBequivalent=0
  powergui : powerlib/powergui  Priority=1  SimulationMode=Discrete  SampleTime=3e-8  frequency=60  Iterations=50  frequencyindice=0  Pbase=100e6  ErrMax=1e-4  UnitsV=kV  UnitsW=MW  buscounter=0  FunctionMessages=off  echomessages=off  EnableUseOfTLC=off  CurrentSourceSwitches=off  DisableSnubberDevices=off  DisableRonSwitches=off  DisableVfSwitches=off  DisplayEquations=off  SolverType=Tustin/Backward Euler (TBE)  Interpol=off  ExternalGateDelay=off  methode=off  Ts=100  x0status=blocks  SPID=off  SwTol=0  HookPort=off  RestoreLinks=warning  ResistiveCurrentMeasurement=off  Frange=[0:2:500]  Ylog=off  Xlog=on  ShowGrid=off  save=off  variable=ZData  structure=0  ZoomFFT=off  StartTime=0.0  cycles=1  DisplayStyle=1  fundamental=60  FreqAxis=off  MaxFrequency=1000  frequencyindicesteady=1  RmsSteady=1  display=off
  PV + ve : PMIOPort  Side=Right
  PV -ve : PMIOPort  Port=2  Side=Right
  wires:
  Demux/2 -> Scope5/2, Boost Converter with Fuzzy Controller/2(PV - I)
  "Temp "/1 -> PV Array/2, Scope2/2
  Boost Converter with Fuzzy Controller/1(Power) -> Scope2/3, Scope/1
  Demux/4 -> Scope5/4
  PV Array/1 -> Demux/1
  IRR 2/1 -> PV Array/1, Scope2/1
  Demux/1 -> Scope5/1, Boost Converter with Fuzzy Controller/1(" PV- V")
  Demux/5 -> Scope5/5
  Demux/3 -> Scope5/3
  Voltage Measurement/1 -> Scope1/1
  connections:
  PV Array/RConn1 -- Boost Converter with Fuzzy Controller/LConn1
  Boost Converter with Fuzzy Controller/RConn1 -- Voltage Measurement/LConn1 -- PV + ve/RConn1
  Boost Converter with Fuzzy Controller/RConn2 -- Voltage Measurement/LConn2 -- PV -ve/RConn1
  PV Array/RConn2 -- Boost Converter with Fuzzy Controller/LConn2

== system FuzzyHYPFWMLI/PV Array 2 ==
  note: Fuzzy Based MPPT Controller for 10 kW PV System
  Demux : Demux  Outputs=5
  IRR 2 : powerlib_extras/Control  Blocks/Timer  t=[0 0.05 0.1 0.15 0.2 ]  e=[250 500 750 1000 1000]
  PV Array : re_lib/Solar/PV Array  Npar=6  Nser=9  PlotType=array @ 25 deg.C & specified irradiances  S_vec="[ 1000  500  100 ]"  Temp_C_vec="[ 45 25  ]"  ModuleName=BP Solar SX3200W  PlotWhenSelected=off  Pm=199.92  Ncell=50  Voc=30.8  Isc=8.7  Vm=24.5  Im=8.16  beta_Voc_pc=-0.33  alpha_Isc_pc=0.1  beta_Voc=-0.10164  alpha_Isc=0.0087  IL=8.7449  I0=1.0576e-10  nI=0.95448  Rsh=190.2563  Rs=0.32982  BAL=off  Tc=1e-6  Tfilter=5e-5
  Scope : Scope
  Scope1 : Scope
  Scope2 : Scope  NumInputPorts=3
  Scope5 : Scope  NumInputPorts=5
  Subsystem2 : Subsystem
  "Temp " : Constant  Value=25
  Voltage Measurement : powerlib/Measurements/Voltage Measurement  PhasorSimulation=off  OutputType=Complex  PSBequivalent=0
  powergui : powerlib/powergui  Priority=1  SimulationMode=Discrete  SampleTime=3e-8  frequency=60  Iterations=50  frequencyindice=0  Pbase=100e6  ErrMax=1e-4  UnitsV=kV  UnitsW=MW  buscounter=0  FunctionMessages=off  echomessages=off  EnableUseOfTLC=off  CurrentSourceSwitches=off  DisableSnubberDevices=off  DisableRonSwitches=off  DisableVfSwitches=off  DisplayEquations=off  SolverType=Tustin/Backward Euler (TBE)  Interpol=off  ExternalGateDelay=off  methode=off  Ts=100  x0status=blocks  SPID=off  SwTol=0  HookPort=off  RestoreLinks=warning  ResistiveCurrentMeasurement=off  Frange=[0:2:500]  Ylog=off  Xlog=on  ShowGrid=off  save=off  variable=ZData  structure=0  ZoomFFT=off  StartTime=0.0  cycles=1  DisplayStyle=1  fundamental=60  FreqAxis=off  MaxFrequency=1000  frequencyindicesteady=1  RmsSteady=1  display=off
  PV + ve : PMIOPort  Side=Right
  PV -ve : PMIOPort  Port=2  Side=Right
  wires:
  Voltage Measurement/1 -> Scope1/1
  Demux/3 -> Scope5/3
  Demux/5 -> Scope5/5
  Demux/1 -> Subsystem2/1(" PV- V"), Scope5/1
  IRR 2/1 -> Scope2/1, PV Array/1
  PV Array/1 -> Demux/1
  Demux/4 -> Scope5/4
  Subsystem2/1(Power) -> Scope/1, Scope2/3
  "Temp "/1 -> Scope2/2, PV Array/2
  Demux/2 -> Subsystem2/2(PV - I), Scope5/2
  connections:
  PV Array/RConn2 -- Subsystem2/LConn2
  PV -ve/RConn1 -- Voltage Measurement/LConn2 -- Subsystem2/RConn2
  PV + ve/RConn1 -- Voltage Measurement/LConn1 -- Subsystem2/RConn1
  PV Array/RConn1 -- Subsystem2/LConn1

== system FuzzyHYPFWMLI/PV Array 3 ==
  note: Fuzzy Based MPPT Controller for 10 kW PV System
  Demux : Demux  Outputs=5
  IRR 2 : powerlib_extras/Control  Blocks/Timer  t=[0 0.05 0.1 0.15 0.2 ]  e=[250 500 750 1000 1000]
  PV Array : re_lib/Solar/PV Array  Npar=6  Nser=9  PlotType=array @ 25 deg.C & specified irradiances  S_vec="[ 1000  500  100 ]"  Temp_C_vec="[ 45 25  ]"  ModuleName=BP Solar SX3200W  PlotWhenSelected=off  Pm=199.92  Ncell=50  Voc=30.8  Isc=8.7  Vm=24.5  Im=8.16  beta_Voc_pc=-0.33  alpha_Isc_pc=0.1  beta_Voc=-0.10164  alpha_Isc=0.0087  IL=8.7449  I0=1.0576e-10  nI=0.95448  Rsh=190.2563  Rs=0.32982  BAL=off  Tc=1e-6  Tfilter=5e-5
  Scope : Scope
  Scope1 : Scope
  Scope2 : Scope  NumInputPorts=3
  Scope5 : Scope  NumInputPorts=5
  Subsystem2 : Subsystem
  "Temp " : Constant  Value=25
  Voltage Measurement : powerlib/Measurements/Voltage Measurement  PhasorSimulation=off  OutputType=Complex  PSBequivalent=0
  powergui : powerlib/powergui  Priority=1  SimulationMode=Discrete  SampleTime=3e-8  frequency=60  Iterations=50  frequencyindice=0  Pbase=100e6  ErrMax=1e-4  UnitsV=kV  UnitsW=MW  buscounter=0  FunctionMessages=off  echomessages=off  EnableUseOfTLC=off  CurrentSourceSwitches=off  DisableSnubberDevices=off  DisableRonSwitches=off  DisableVfSwitches=off  DisplayEquations=off  SolverType=Tustin/Backward Euler (TBE)  Interpol=off  ExternalGateDelay=off  methode=off  Ts=100  x0status=blocks  SPID=off  SwTol=0  HookPort=off  RestoreLinks=warning  ResistiveCurrentMeasurement=off  Frange=[0:2:500]  Ylog=off  Xlog=on  ShowGrid=off  save=off  variable=ZData  structure=0  ZoomFFT=off  StartTime=0.0  cycles=1  DisplayStyle=1  fundamental=60  FreqAxis=off  MaxFrequency=1000  frequencyindicesteady=1  RmsSteady=1  display=off
  PV + ve : PMIOPort  Side=Right
  PV -ve : PMIOPort  Port=2  Side=Right
  wires:
  Demux/2 -> Scope5/2, Subsystem2/2(PV - I)
  "Temp "/1 -> PV Array/2, Scope2/2
  Subsystem2/1(Power) -> Scope2/3, Scope/1
  Demux/4 -> Scope5/4
  PV Array/1 -> Demux/1
  IRR 2/1 -> PV Array/1, Scope2/1
  Demux/1 -> Scope5/1, Subsystem2/1(" PV- V")
  Demux/5 -> Scope5/5
  Demux/3 -> Scope5/3
  Voltage Measurement/1 -> Scope1/1
  connections:
  PV Array/RConn1 -- Subsystem2/LConn1
  Subsystem2/RConn1 -- Voltage Measurement/LConn1 -- PV + ve/RConn1
  Subsystem2/RConn2 -- Voltage Measurement/LConn2 -- PV -ve/RConn1
  PV Array/RConn2 -- Subsystem2/LConn2

== system FuzzyHYPFWMLI/VSC Control2 ==
  note: VSC Main Controller
  Vabc_prim : Inport  PortDimensions=3
  Iabc_prim : Inport  Port=2  PortDimensions=3
  Vdc_mes : Inport  Port=3  PortDimensions=1
  Current Regulator : Subsystem
  Iq_ref : Constant  Value=0
  Mux : Mux  Inputs=2
  PLL & Measurements : Subsystem
  PWM Generator (2-Level) : powerlib_meascontrol/Pulse & Signal Generators/PWM Generator (2-Level)  ModulatorType=Three-phase bridge (6 pulses)  ModulatorMode=Unsynchronized  Fc=27*50  Pc=90  nF=27  MinMax="[ -1  1 ]"  SamplingTechnique=Natural  ModulatingSignals=off  m=0.8  Freq=60  Phase=0  Ts=0  ShowCarrierOutport=off
      settings: SourceProductName=Simscape Power Systems
  Uabc_ref Generation max (m) = 1 : Subsystem
  Unit Delay : UnitDelay  SampleTime=1e-6  HasFrameUpgradeWarning=on
  VDC Regulator : Subsystem
  Vdc_ref1 : Constant  Value=Vdc_ref
  Pulses : Outport  VectorParamsAs1DForOutWhenUnconnected=off
  wires:
  VDC Regulator/1(Id_ref) -> Mux/1
  PLL & Measurements/1(wt) -> Uabc_ref Generation max (m) = 1/1(wt)
  Current Regulator/1(VdVq_conv) -> Uabc_ref Generation max (m) = 1/2(VdVq_conv)
  Iq_ref/1 -> Mux/2
  Mux/1 -> Current Regulator/3(IdIq_ref)
  PLL & Measurements/3(IdIq_prim) -> Current Regulator/2(IdIq_mes)
  PLL & Measurements/2(VdVq_prim) -> Current Regulator/1(VdVq_mes)
  Vdc_mes/1 -> VDC Regulator/1(Vdc_mes)
  Vabc_prim/1 -> PLL & Measurements/1(Vabc_prim)
  Iabc_prim/1 -> PLL & Measurements/2(Iabc_prim)
  Unit Delay/1 -> PWM Generator (2-Level)/1
  PWM Generator (2-Level)/1 -> Pulses/1
  Uabc_ref Generation max (m) = 1/1(Uabc_ref) -> Unit Delay/1
  Vdc_ref1/1 -> VDC Regulator/2(Vdc_ref)
